simulink model "TestBench"  (Simulink 7.6)
settings: Solver=ode45  StartTime=0.0  StopTime=100  RelTol=1e-3
InitFcn:
  | TestBench_datastruct
  | SCAP
undefined symbols (not defined in the file): determiningBonds, sigbuilder_block
(part 1 of 2)
settings Model: Creator=Zsolt  LastModifiedBy=Zsolt
settings HardwareCC: TargetIntDivRoundTo=Zero  TargetEndianess=LittleEndian  TargetHWDeviceType=MATLAB Host  ProdEqTarget=off
settings RTWCC: SystemTargetFile=rsim.tlc  TemplateMakefile=rsim_default_tmf  Description=Rapid Simulation Target  ProcessScript=rsim_make_rtw_hook
settings RSimTargetCC: TargetFunctionLibrary=ANSI_C  ERTMultiwordTypeDef=System defined  ERTCodeCoverageTool=None  ERTMultiwordLength=256  IsPILTarget=off  EnableShiftOperators=on  PortableWordSizes=off

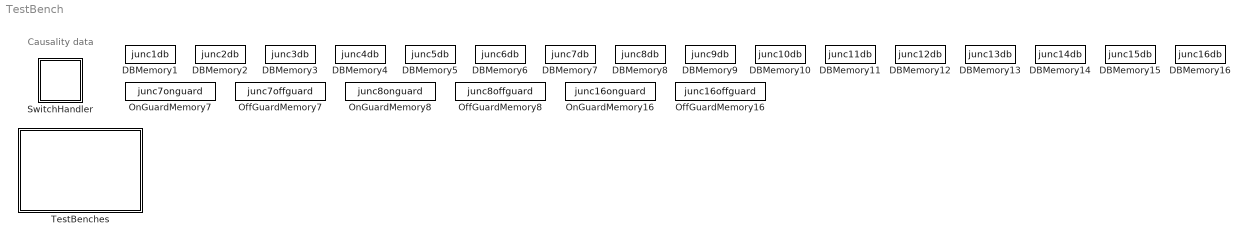
== system TestBench ==
  note: Causality data
  DBMemory1 : DataStoreMemory  DataStoreName=junc1db  InitialValue=determiningBonds(1)
  DBMemory10 : DataStoreMemory  DataStoreName=junc10db  InitialValue=determiningBonds(10)
  DBMemory11 : DataStoreMemory  DataStoreName=junc11db  InitialValue=determiningBonds(11)
  DBMemory12 : DataStoreMemory  DataStoreName=junc12db  InitialValue=determiningBonds(12)
  DBMemory13 : DataStoreMemory  DataStoreName=junc13db  InitialValue=determiningBonds(13)
  DBMemory14 : DataStoreMemory  DataStoreName=junc14db  InitialValue=determiningBonds(14)
  DBMemory15 : DataStoreMemory  DataStoreName=junc15db  InitialValue=determiningBonds(15)
  DBMemory16 : DataStoreMemory  DataStoreName=junc16db  InitialValue=determiningBonds(16)
  DBMemory2 : DataStoreMemory  DataStoreName=junc2db  InitialValue=determiningBonds(2)
  DBMemory3 : DataStoreMemory  DataStoreName=junc3db  InitialValue=determiningBonds(3)
  DBMemory4 : DataStoreMemory  DataStoreName=junc4db  InitialValue=determiningBonds(4)
  DBMemory5 : DataStoreMemory  DataStoreName=junc5db  InitialValue=determiningBonds(5)
  DBMemory6 : DataStoreMemory  DataStoreName=junc6db  InitialValue=determiningBonds(6)
  DBMemory7 : DataStoreMemory  DataStoreName=junc7db  InitialValue=determiningBonds(7)
  DBMemory8 : DataStoreMemory  DataStoreName=junc8db  InitialValue=determiningBonds(8)
  DBMemory9 : DataStoreMemory  DataStoreName=junc9db  InitialValue=determiningBonds(9)
  OffGuardMemory16 : DataStoreMemory  DataStoreName=junc16offguard
  OffGuardMemory7 : DataStoreMemory  DataStoreName=junc7offguard
  OffGuardMemory8 : DataStoreMemory  DataStoreName=junc8offguard
  OnGuardMemory16 : DataStoreMemory  DataStoreName=junc16onguard
  OnGuardMemory7 : DataStoreMemory  DataStoreName=junc7onguard
  OnGuardMemory8 : DataStoreMemory  DataStoreName=junc8onguard
  SwitchHandler : Subsystem
  TestBenches : Subsystem

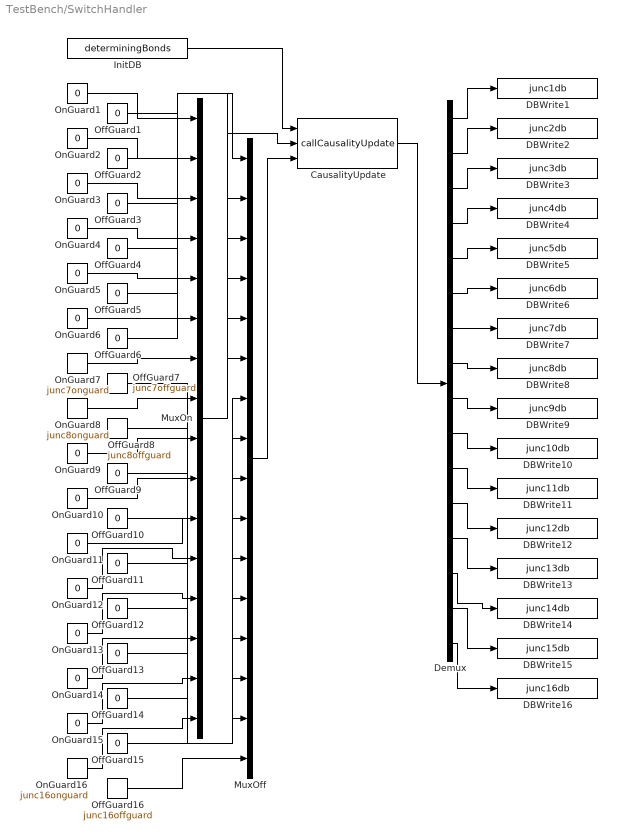
== system TestBench/SwitchHandler ==
  CausalityUpdate : S-Function  FunctionName=callCausalityUpdate  Parameters=16  EnableBusSupport=off
  DBWrite1 : DataStoreWrite  DataStoreName=junc1db
  DBWrite10 : DataStoreWrite  DataStoreName=junc10db
  DBWrite11 : DataStoreWrite  DataStoreName=junc11db
  DBWrite12 : DataStoreWrite  DataStoreName=junc12db
  DBWrite13 : DataStoreWrite  DataStoreName=junc13db
  DBWrite14 : DataStoreWrite  DataStoreName=junc14db
  DBWrite15 : DataStoreWrite  DataStoreName=junc15db
  DBWrite16 : DataStoreWrite  DataStoreName=junc16db
  DBWrite2 : DataStoreWrite  DataStoreName=junc2db
  DBWrite3 : DataStoreWrite  DataStoreName=junc3db
  DBWrite4 : DataStoreWrite  DataStoreName=junc4db
  DBWrite5 : DataStoreWrite  DataStoreName=junc5db
  DBWrite6 : DataStoreWrite  DataStoreName=junc6db
  DBWrite7 : DataStoreWrite  DataStoreName=junc7db
  DBWrite8 : DataStoreWrite  DataStoreName=junc8db
  DBWrite9 : DataStoreWrite  DataStoreName=junc9db
  Demux : Demux  Outputs=16
  InitDB : Constant  Value=determiningBonds
  MuxOff : Mux  Inputs=16
  MuxOn : Mux  Inputs=16
  OffGuard{1..6,9..15} (13 alike) : Constant  Value=0
  OffGuard16 : DataStoreRead  DataStoreName=junc16offguard  SampleTime=0
  OffGuard7 : DataStoreRead  DataStoreName=junc7offguard  SampleTime=0
  OffGuard8 : DataStoreRead  DataStoreName=junc8offguard  SampleTime=0
  OnGuard{1..6,9..15} (13 alike) : Constant  Value=0
  OnGuard16 : DataStoreRead  DataStoreName=junc16onguard  SampleTime=0
  OnGuard7 : DataStoreRead  DataStoreName=junc7onguard  SampleTime=0
  OnGuard8 : DataStoreRead  DataStoreName=junc8onguard  SampleTime=0
  wires:
  OnGuard1/1 -> MuxOn/1
  OffGuard1/1 -> MuxOff/1
  Demux/1 -> DBWrite1/1
  OnGuard2/1 -> MuxOn/2
  OffGuard2/1 -> MuxOff/2
  Demux/2 -> DBWrite2/1
  OnGuard3/1 -> MuxOn/3
  OffGuard3/1 -> MuxOff/3
  Demux/3 -> DBWrite3/1
  OnGuard4/1 -> MuxOn/4
  OffGuard4/1 -> MuxOff/4
  Demux/4 -> DBWrite4/1
  OnGuard5/1 -> MuxOn/5
  OffGuard5/1 -> MuxOff/5
  Demux/5 -> DBWrite5/1
  OnGuard6/1 -> MuxOn/6
  OffGuard6/1 -> MuxOff/6
  Demux/6 -> DBWrite6/1
  OnGuard7/1 -> MuxOn/7
  OffGuard7/1 -> MuxOff/7
  Demux/7 -> DBWrite7/1
  OnGuard8/1 -> MuxOn/8
  OffGuard8/1 -> MuxOff/8
  Demux/8 -> DBWrite8/1
  OnGuard9/1 -> MuxOn/9
  OffGuard9/1 -> MuxOff/9
  Demux/9 -> DBWrite9/1
  OnGuard10/1 -> MuxOn/10
  OffGuard10/1 -> MuxOff/10
  Demux/10 -> DBWrite10/1
  OnGuard11/1 -> MuxOn/11
  OffGuard11/1 -> MuxOff/11
  Demux/11 -> DBWrite11/1
  OnGuard12/1 -> MuxOn/12
  OffGuard12/1 -> MuxOff/12
  Demux/12 -> DBWrite12/1
  OnGuard13/1 -> MuxOn/13
  OffGuard13/1 -> MuxOff/13
  Demux/13 -> DBWrite13/1
  OnGuard14/1 -> MuxOn/14
  OffGuard14/1 -> MuxOff/14
  Demux/14 -> DBWrite14/1
  OnGuard15/1 -> MuxOn/15
  OffGuard15/1 -> MuxOff/15
  Demux/15 -> DBWrite15/1
  OnGuard16/1 -> MuxOn/16
  OffGuard16/1 -> MuxOff/16
  Demux/16 -> DBWrite16/1
  InitDB/1 -> CausalityUpdate/1
  MuxOn/1 -> CausalityUpdate/2
  MuxOff/1 -> CausalityUpdate/3
  CausalityUpdate/1 -> Demux/1

== system TestBench/TestBenches ==
  V_EngISGTest_experiments : Subsystem

== system TestBench/TestBenches/V_EngISGTest_experiments ==
  EngineISG : Subsystem
  RotationalLoad : Subsystem
  ThrottleScenario : Subsystem
  wires:
  EngineISG/1(RotationalPowerPort_1_OUT_5) -> RotationalLoad/1(Rotational Power Port_1_IN_5)
  RotationalLoad/1(Rotational Power Port_1_OUT_5) -> EngineISG/1(RotationalPowerPort_1_IN_5)
  ThrottleScenario/1(Mode) -> EngineISG/5(Mode)
  ThrottleScenario/2(DieselDemand) -> EngineISG/3(Throttle)
  ThrottleScenario/3(ElectDemand) -> EngineISG/4(EP_Demand)

== system TestBench/TestBenches/V_EngISGTest_experiments/EngineISG ==
  RotationalPowerPort_1_IN_5 : Inport
  AddlLoad : Inport  Port=2
  Throttle : Inport  Port=3
  EP_Demand : Inport  Port=4
  Mode : Inport  Port=5
  Battery : Subsystem
  Diesel_Engine : Subsystem
  ISG : Subsystem
  PowerController : Subsystem
  RotationalPowerPort_1_OUT_5 : Outport
  wires:
  Diesel_Engine/1(OutputShaft_1_OUT_2) -> ISG/1(EngSide_1_IN_2)
  ISG/1(EngSide_1_OUT_2) -> Diesel_Engine/1(OutputShaft_1_IN_2)
  Battery/1(Pwr_1_OUT_3) -> PowerController/1(Batt_In_1_IN_3)
  PowerController/1(Batt_In_1_OUT_3) -> Battery/1(Pwr_1_IN_3)
  ISG/2(TransSide_1_OUT_5) -> RotationalPowerPort_1_OUT_5/1
  RotationalPowerPort_1_IN_5/1 -> ISG/2(TransSide_1_IN_5)
  PowerController/2(ISG_Out_1_OUT_7) -> ISG/3(ElectricalPowerPort_1_IN_7)
  ISG/3(ElectricalPowerPort_1_OUT_7) -> PowerController/2(ISG_Out_1_IN_7)
  Throttle/1 -> Diesel_Engine/3(Throttle)
  AddlLoad/1 -> Diesel_Engine/2(Additional_Load)
  Mode/1 -> Battery/2(Mode)
  Battery/2(BatteryVoltage) -> PowerController/4(BattVoltage)
  EP_Demand/1 -> PowerController/5(E_Power_Demand)
  ISG/6(ISG_EngVoltage) -> PowerController/3(ISGVoltage)

== system TestBench/TestBenches/V_EngISGTest_experiments/RotationalLoad ==
  Rotational Power Port_1_IN_5 : Inport
  Load : Constant  Value=3000
  ResistiveLoad : Subsystem
  Targthrottle : Constant
  Rotational Power Port_1_OUT_5 : Outport
  AddLoad : Outport  Port=2
  Throttle : Outport  Port=3
  wires:
  ResistiveLoad/1(MechanicalRPort_1_OUT_5) -> Rotational Power Port_1_OUT_5/1
  Rotational Power Port_1_IN_5/1 -> ResistiveLoad/1(MechanicalRPort_1_IN_5)
  Targthrottle/1 -> Throttle/1
  Load/1 -> AddLoad/1

== system TestBench/TestBenches/V_EngISGTest_experiments/ThrottleScenario ==
  BGDriver : Subsystem
  Mode : Outport
  DieselDemand : Outport  Port=2
  ElectDemand : Outport  Port=3
  wires:
  BGDriver/3(Mode) -> Mode/1
  BGDriver/1(MechPwr) -> DieselDemand/1
  BGDriver/2(ElecPwr) -> ElectDemand/1

== system TestBench/TestBenches/V_EngISGTest_experiments/EngineISG/Battery ==
  Pwr_1_IN_3 : Inport
  Mode : Inport  Port=2
  Battery : Subsystem
  Pwr_1_OUT_3 : Outport
  BatteryVoltage : Outport  Port=2
  wires:
  Battery/1(Pwr_1_OUT_3) -> Pwr_1_OUT_3/1
  Pwr_1_IN_3/1 -> Battery/1(Pwr_1_IN_3)
  Battery/2(Battery_Voltage) -> BatteryVoltage/1
  Mode/1 -> Battery/2(Mode)

== system TestBench/TestBenches/V_EngISGTest_experiments/EngineISG/Diesel_Engine ==
  OutputShaft_1_IN_2 : Inport
  Additional_Load : Inport  Port=2
  Throttle : Inport  Port=3
  Diesel_Engine : Subsystem
  MaxPower : Constant  Value=300000
  MaxTorque : Constant  Value=2000
  OutputShaft_1_OUT_2 : Outport
  Angular_Velocity : Outport  Port=2
  wires:
  Diesel_Engine/1(Out_1_OUT_2) -> OutputShaft_1_OUT_2/1
  OutputShaft_1_IN_2/1 -> Diesel_Engine/1(Out_1_IN_2)
  Diesel_Engine/2(Angular_Velocity) -> Angular_Velocity/1
  Additional_Load/1 -> Diesel_Engine/5(Additional_Load)
  Throttle/1 -> Diesel_Engine/2(Throttle)
  MaxTorque/1 -> Diesel_Engine/3(torqueMax)
  MaxPower/1 -> Diesel_Engine/4(MaxPower)

== system TestBench/TestBenches/V_EngISGTest_experiments/EngineISG/ISG ==
  EngSide_1_IN_2 : Inport
  TransSide_1_IN_5 : Inport  Port=2
  ElectricalPowerPort_1_IN_7 : Inport  Port=3
  ISG_BG : Subsystem
  ISG_Gain : Constant  Value=0.05
  EngSide_1_OUT_2 : Outport
  TransSide_1_OUT_5 : Outport  Port=2
  ElectricalPowerPort_1_OUT_7 : Outport  Port=3
  AngularVelocity : Outport  Port=4
  AddedTorque : Outport  Port=5
  ISG_EngVoltage : Outport  Port=6
  wires:
  ISG_BG/1(EngineSide_1_OUT_2) -> EngSide_1_OUT_2/1
  EngSide_1_IN_2/1 -> ISG_BG/1(EngineSide_1_IN_2)
  ISG_BG/2(TransmissionSide_1_OUT_5) -> TransSide_1_OUT_5/1
  TransSide_1_IN_5/1 -> ISG_BG/2(TransmissionSide_1_IN_5)
  ISG_BG/3(Electrical_1_OUT_7) -> ElectricalPowerPort_1_OUT_7/1
  ElectricalPowerPort_1_IN_7/1 -> ISG_BG/3(Electrical_1_IN_7)
  ISG_BG/4(ISG_AngularVelocity) -> AngularVelocity/1
  ISG_BG/5(ISG_Torque) -> AddedTorque/1
  ISG_BG/6(InV) -> ISG_EngVoltage/1
  ISG_Gain/1 -> ISG_BG/4(ISG_GainInput)

== system TestBench/TestBenches/V_EngISGTest_experiments/EngineISG/PowerController ==
  Batt_In_1_IN_3 : Inport
  ISG_Out_1_IN_7 : Inport  Port=2
  ISGVoltage : Inport  Port=3
  BattVoltage : Inport  Port=4
  E_Power_Demand : Inport  Port=5
  PowerCtrlBG : Subsystem
  Batt_In_1_OUT_3 : Outport
  ISG_Out_1_OUT_7 : Outport  Port=2
  wires:
  PowerCtrlBG/1(Batt_Input_1_OUT_3) -> Batt_In_1_OUT_3/1
  Batt_In_1_IN_3/1 -> PowerCtrlBG/1(Batt_Input_1_IN_3)
  PowerCtrlBG/2(Power_Output_1_OUT_7) -> ISG_Out_1_OUT_7/1
  ISG_Out_1_IN_7/1 -> PowerCtrlBG/2(Power_Output_1_IN_7)
  E_Power_Demand/1 -> PowerCtrlBG/5(Demand)
  BattVoltage/1 -> PowerCtrlBG/4(BattVoltage)
  ISGVoltage/1 -> PowerCtrlBG/3(ISGVoltage)

== system TestBench/TestBenches/V_EngISGTest_experiments/RotationalLoad/ResistiveLoad ==
  MechanicalRPort_1_IN_5 : Inport
  InertialLoad : Subsystem  mask{I=10, IC=0}
      mask prompts: I "Value of I:"; IC "Initial Condition:"
      mask Display: image(imread('I.png','BackgroundColor',[1 1 1]))
  Load_w : Scope
  ResistiveLoad2 : Subsystem  mask{R=1.5}
      mask prompts: R "Value of R:"
      mask Display: image(imread('R.png','BackgroundColor',[1 1 1]))
  Series : Subsystem
      mask Display: image(imread('1.png','BackgroundColor',[1 1 1]))
  zed1 : Subsystem
      mask Display: image(imread('0.png','BackgroundColor',[1 1 1]))
  MechanicalRPort_1_OUT_5 : Outport
  wires:
  zed1/2(y(2)) -> Series/2(u(2))
  Series/2(y(2)) -> zed1/2(u(2))
  Series/1(y(1)) -> ResistiveLoad2/1(In)
  ResistiveLoad2/1(Out) -> Series/1(u(1))
  Series/3(y(3)) -> InertialLoad/1(E)
  InertialLoad/1(F) -> Series/3(u(3))
  zed1/1(y(1)) -> MechanicalRPort_1_OUT_5/1
  MechanicalRPort_1_IN_5/1 -> zed1/1(u(1))
  Series/4(O) -> Load_w/1

== system TestBench/TestBenches/V_EngISGTest_experiments/ThrottleScenario/BGDriver ==
  SimulinkModel : Subsystem
  MechPwr : Outport
  ElecPwr : Outport  Port=2
  Mode : Outport  Port=3
  wires:
  SimulinkModel/1(Mode) -> Mode/1
  SimulinkModel/2(Mech_Pwr) -> MechPwr/1
  SimulinkModel/3(Elect_Pwr) -> ElecPwr/1

== system TestBench/TestBenches/V_EngISGTest_experiments/EngineISG/Battery/Battery ==
  Pwr_1_IN_3 : Inport
  Mode : Inport  Port=2
  C_battery : Subsystem  mask{C=100, IC=24}
      mask prompts: C "Value of C:"; IC "Initial Condition:"
      mask Display: image(imread('C.png','BackgroundColor',[1 1 1]))
  Current_Battery : Scope
  De_batt_voltage : Subsystem  TreatAsAtomicUnit=on
  R_battery : Subsystem  mask{R=0.01}
      mask prompts: R "Value of R:"
      mask Display: image(imread('R.png','BackgroundColor',[1 1 1]))
  Voltage_Battery : Scope
  oj1 : Subsystem
      mask Display: image(imread('1.png','BackgroundColor',[1 1 1]))
  zj2 : Subsystem
      mask Display: image(imread('0.png','BackgroundColor',[1 1 1]))
  Pwr_1_OUT_3 : Outport
  Battery_Voltage : Outport  Port=2
  wires:
  oj1/2(y(2)) -> R_battery/1(In)
  R_battery/1(Out) -> oj1/2(u(2))
  zj2/1(y(1)) -> oj1/3(u(3))
  oj1/3(y(3)) -> zj2/1(u(1))
  zj2/2(y(2)) -> C_battery/1(F)
  C_battery/1(E) -> zj2/2(u(2))
  oj1/1(y(1)) -> Pwr_1_OUT_3/1
  Pwr_1_IN_3/1 -> oj1/1(u(1))
  zj2/3(O) -> Voltage_Battery/1, De_batt_voltage/1(E_In)
  Mode/1 -> oj1/4(u(4))
  De_batt_voltage/1(E_Out) -> Battery_Voltage/1
  oj1/4(O) -> Current_Battery/1

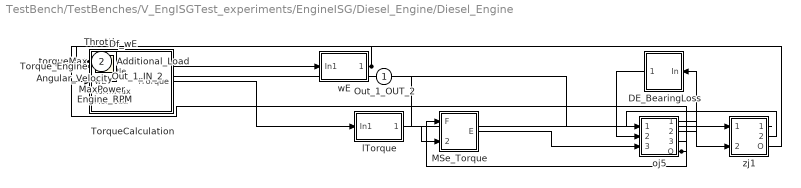
== system TestBench/TestBenches/V_EngISGTest_experiments/EngineISG/Diesel_Engine/Diesel_Engine ==
  Out_1_IN_2 : Inport
  Throttle : Inport  Port=2
  torqueMax : Inport  Port=3
  MaxPower : Inport  Port=4
  Additional_Load : Inport  Port=5
  DE_BearingLoss : Subsystem  mask{R=0.01}
      mask prompts: R "Value of R:"
      mask Display: image(imread('R.png','BackgroundColor',[1 1 1]))
  Df_wE : Subsystem  TreatAsAtomicUnit=on
  Engine_RPM : Scope
  MSe_Torque : Subsystem
      mask Display: image(imread('MSe.png','BackgroundColor',[1 1 1]))
  TorqueCalculation : Stateflow chart  TreatAsAtomicUnit=on
  Torque_Engine : Scope
  lTorque : Subsystem  TreatAsAtomicUnit=on
  oj5 : Subsystem
      mask Display: image(imread('1.png','BackgroundColor',[1 1 1]))
  wE : Subsystem  TreatAsAtomicUnit=on
  zj1 : Subsystem
      mask Display: image(imread('0.png','BackgroundColor',[1 1 1]))
  Out_1_OUT_2 : Outport
  Angular_Velocity : Outport  Port=2
  wires:
  oj5/1(y(1)) -> zj1/2(u(2))
  zj1/2(y(2)) -> oj5/1(u(1))
  oj5/2(y(2)) -> DE_BearingLoss/1(In)
  DE_BearingLoss/1(Out) -> oj5/2(u(2))
  MSe_Torque/1(E) -> oj5/3(u(3))
  oj5/3(y(3)) -> MSe_Torque/1(F)
  zj1/1(y(1)) -> Out_1_OUT_2/1
  Out_1_IN_2/1 -> zj1/1(u(1))
  TorqueCalculation/1(lTorque) -> lTorque/1(In1)
  zj1/3(O) -> Torque_Engine/1
  lTorque/1(Out1) -> MSe_Torque/2(Se Value)
  Throttle/1 -> TorqueCalculation/2(Throttle)
  torqueMax/1 -> TorqueCalculation/4(torqueMax)
  MaxPower/1 -> TorqueCalculation/1(MaxPower)
  Additional_Load/1 -> TorqueCalculation/5(Additional_Load)
  Df_wE/1(F_Out) -> wE/1(In1)
  oj5/4(O) -> Df_wE/1(F_In), Engine_RPM/1
  wE/1(Out1) -> TorqueCalculation/3(wE), Angular_Velocity/1

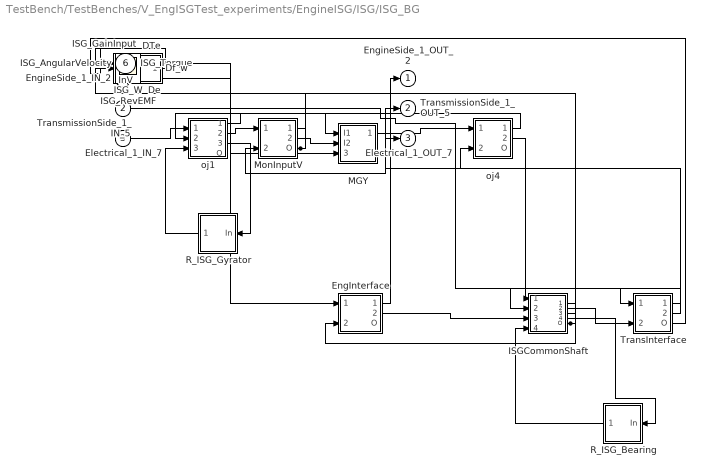
== system TestBench/TestBenches/V_EngISGTest_experiments/EngineISG/ISG/ISG_BG ==
  EngineSide_1_IN_2 : Inport
  TransmissionSide_1_IN_5 : Inport  Port=2
  Electrical_1_IN_7 : Inport  Port=3
  ISG_GainInput : Inport  Port=4
  DTe : Subsystem  TreatAsAtomicUnit=on
  De : Subsystem  TreatAsAtomicUnit=on
  Df_w : Subsystem  TreatAsAtomicUnit=on
  EngInterface : Subsystem
      mask Display: image(imread('0.png','BackgroundColor',[1 1 1]))
  ISGCommonShaft : Subsystem
      mask Display: image(imread('1.png','BackgroundColor',[1 1 1]))
  ISG_RevEMF : Scope
  ISG_W : Scope
  MGY : Subsystem
      mask Display: image(imread('MGY.png','BackgroundColor',[1 1 1]))
  MonInputV : Subsystem
      mask Display: image(imread('0.png','BackgroundColor',[1 1 1]))
  R_ISG_Bearing : Subsystem  mask{R=0.01}
      mask prompts: R "Value of R:"
      mask Display: image(imread('R.png','BackgroundColor',[1 1 1]))
  R_ISG_Gyrator : Subsystem  mask{R=0.01}
      mask prompts: R "Value of R:"
      mask Display: image(imread('R.png','BackgroundColor',[1 1 1]))
  TransInterface : Subsystem
      mask Display: image(imread('0.png','BackgroundColor',[1 1 1]))
  oj1 : Subsystem
      mask Display: image(imread('1.png','BackgroundColor',[1 1 1]))
  oj4 : Subsystem
      mask Display: image(imread('1.png','BackgroundColor',[1 1 1]))
  EngineSide_1_OUT_2 : Outport
  TransmissionSide_1_OUT_5 : Outport  Port=2
  Electrical_1_OUT_7 : Outport  Port=3
  ISG_AngularVelocity : Outport  Port=4
  ISG_Torque : Outport  Port=5
  InV : Outport  Port=6
  wires:
  EngInterface/2(y(2)) -> ISGCommonShaft/3(u(3))
  ISGCommonShaft/3(y(3)) -> EngInterface/2(u(2))
  oj1/2(y(2)) -> MonInputV/1(u(1))
  MonInputV/1(y(1)) -> oj1/2(u(2))
  oj1/3(y(3)) -> R_ISG_Gyrator/1(In)
  R_ISG_Gyrator/1(Out) -> oj1/3(u(3))
  MGY/1(O1) -> oj4/1(u(1))
  oj4/1(y(1)) -> MGY/1(I1)
  oj4/2(y(2)) -> ISGCommonShaft/1(u(1))
  ISGCommonShaft/1(y(1)) -> oj4/2(u(2))
  ISGCommonShaft/2(y(2)) -> TransInterface/2(u(2))
  TransInterface/2(y(2)) -> ISGCommonShaft/2(u(2))
  ISGCommonShaft/4(y(4)) -> R_ISG_Bearing/1(In)
  R_ISG_Bearing/1(Out) -> ISGCommonShaft/4(u(4))
  MonInputV/2(y(2)) -> MGY/2(I2)
  MGY/2(O2) -> MonInputV/2(u(2))
  EngInterface/1(y(1)) -> EngineSide_1_OUT_2/1
  EngineSide_1_IN_2/1 -> EngInterface/1(u(1))
  TransInterface/1(y(1)) -> TransmissionSide_1_OUT_5/1
  TransmissionSide_1_IN_5/1 -> TransInterface/1(u(1))
  oj1/1(y(1)) -> Electrical_1_OUT_7/1
  Electrical_1_IN_7/1 -> oj1/1(u(1))
  Df_w/1(F_Out) -> ISG_AngularVelocity/1
  TransInterface/3(O) -> De/1(E_In)
  ISGCommonShaft/5(O) -> Df_w/1(F_In), ISG_W/1
  De/1(E_Out) -> ISG_Torque/1
  DTe/1(E_Out) -> InV/1
  MonInputV/3(O) -> DTe/1(E_In), ISG_RevEMF/1
  ISG_GainInput/1 -> MGY/3(GY Value)

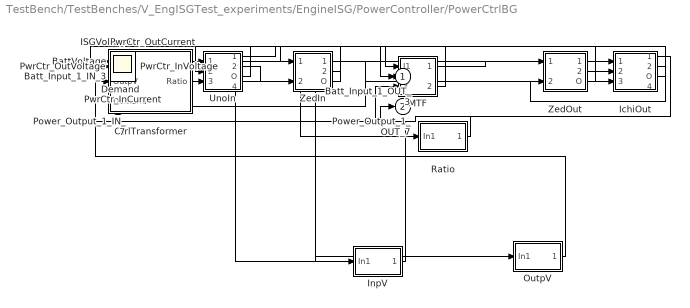
== system TestBench/TestBenches/V_EngISGTest_experiments/EngineISG/PowerController/PowerCtrlBG ==
  Batt_Input_1_IN_3 : Inport
  Power_Output_1_IN_7 : Inport  Port=2
  ISGVoltage : Inport  Port=3
  BattVoltage : Inport  Port=4
  Demand : Inport  Port=5
  CtrlTransformer : Stateflow chart  TreatAsAtomicUnit=on
  IchiOut : Subsystem
      mask Display: image(imread('1.png','BackgroundColor',[1 1 1]))
  InpV : Subsystem  TreatAsAtomicUnit=on
  MTF : Subsystem
      mask Display: image(imread('MTF.png','BackgroundColor',[1 1 1]))
  OutpV : Subsystem  TreatAsAtomicUnit=on
  PwrCtr_InCurrent : Scope
  PwrCtr_InVoltage : Scope
  PwrCtr_OutCurrent : Scope
  PwrCtr_OutVoltage : Scope
  Ratio : Subsystem  TreatAsAtomicUnit=on
  UnoIn : Subsystem
      mask Display: image(imread('1.png','BackgroundColor',[1 1 1]))
  ZedIn : Subsystem
      mask Display: image(imread('0.png','BackgroundColor',[1 1 1]))
  ZedOut : Subsystem
      mask Display: image(imread('0.png','BackgroundColor',[1 1 1]))
  Batt_Input_1_OUT_3 : Outport
  Power_Output_1_OUT_7 : Outport  Port=2
  wires:
  UnoIn/2(y(2)) -> ZedIn/2(u(2))
  ZedIn/2(y(2)) -> UnoIn/2(u(2))
  MTF/1(O1) -> ZedOut/1(u(1))
  ZedOut/1(y(1)) -> MTF/1(I1)
  ZedOut/2(y(2)) -> IchiOut/2(u(2))
  IchiOut/2(y(2)) -> ZedOut/2(u(2))
  ZedIn/1(y(1)) -> MTF/2(I2)
  MTF/2(O2) -> ZedIn/1(u(1))
  UnoIn/1(y(1)) -> Batt_Input_1_OUT_3/1
  Batt_Input_1_IN_3/1 -> UnoIn/1(u(1))
  IchiOut/1(y(1)) -> Power_Output_1_OUT_7/1
  Power_Output_1_IN_7/1 -> IchiOut/1(u(1))
  ISGVoltage/1 -> OutpV/1(In1)
  BattVoltage/1 -> InpV/1(In1)
  InpV/1(Out1) -> CtrlTransformer/1(InpV)
  UnoIn/3(O) -> PwrCtr_InCurrent/1
  Demand/1 -> UnoIn/3(u(3)), IchiOut/3(u(3)), CtrlTransformer/3(Demand)
  ZedIn/3(O) -> PwrCtr_InVoltage/1
  OutpV/1(Out1) -> CtrlTransformer/2(OutpV)
  IchiOut/3(O) -> PwrCtr_OutCurrent/1
  ZedOut/3(O) -> PwrCtr_OutVoltage/1
  Ratio/1(Out1) -> MTF/3(TF Value)
  CtrlTransformer/1(Ratio) -> Ratio/1(In1)

== system TestBench/TestBenches/V_EngISGTest_experiments/RotationalLoad/ResistiveLoad/InertialLoad ==
  E : Inport
  Inductance : Constant  Value=I
  InitialCondition : Constant  Value=IC
  Initialization : InitialCondition  Value=IC
  Integrator : Integrator  InitialConditionSource=external
  Product1 : Product  SaturateOnIntegerOverflow=on  RndMeth=Zero  InputSameDT=on  OutDataTypeStr=Inherit: Same as first input
  Product2 : Product  SaturateOnIntegerOverflow=on  RndMeth=Zero  InputSameDT=on  OutDataTypeStr=Inherit: Same as first input
  Reciprocal : Math  Operator=reciprocal  SaturateOnIntegerOverflow=on
  F : Outport
  p : Outport  Port=2
  wires:
  E/1 -> Integrator/1
  InitialCondition/1 -> Initialization/1
  Initialization/1 -> Product1/1
  Inductance/1 -> Reciprocal/1, Product1/2
  Product1/1 -> Integrator/2
  Integrator/1 -> Product2/1, p/1
  Reciprocal/1 -> Product2/2
  Product2/1 -> F/1

== system TestBench/TestBenches/V_EngISGTest_experiments/RotationalLoad/ResistiveLoad/ResistiveLoad2 ==
  In : Inport
  Bond : Constant
  Computing R : Subsystem
  JuncDB : Constant  Value=3
  Junction Type : Constant
  Resistor Value : Constant  Value=R
  Out : Outport
  wires:
  In/1 -> Computing R/1(In1)
  Resistor Value/1 -> Computing R/2(R)
  JuncDB/1 -> Computing R/3(JuncDB)
  Bond/1 -> Computing R/4(Bond)
  Junction Type/1 -> Computing R/5(Junction Type)
  Computing R/1(Out1) -> Out/1

== system TestBench/TestBenches/V_EngISGTest_experiments/RotationalLoad/ResistiveLoad/Series ==
  u(1) : Inport
  u(2) : Inport  Port=2
  u(3) : Inport  Port=3
  Adder : Sum  Inputs=+-  SaturateOnIntegerOverflow=on  InputSameDT=on  OutDataTypeStr=Inherit: Same as first input
  Gain : Gain  Gain=-1  SaturateOnIntegerOverflow=on  OutDataTypeStr=Inherit: Same as input  ParamDataTypeStr=Inherit: Same as input
  y(1) : Outport
  y(2) : Outport  Port=2
  y(3) : Outport  Port=3
  O : Outport  Port=4
  wires:
  Adder/1 -> Gain/1
  u(3)/1 -> y(1)/1, y(2)/1, O/1
  u(1)/1 -> Adder/1
  u(2)/1 -> Adder/2
  Gain/1 -> y(3)/1

== system TestBench/TestBenches/V_EngISGTest_experiments/RotationalLoad/ResistiveLoad/zed1 ==
  u(1) : Inport
  u(2) : Inport  Port=2
  Adder : Sum  Inputs=+  SaturateOnIntegerOverflow=on  InputSameDT=on  OutDataTypeStr=Inherit: Same as first input
  Gain : Gain  SaturateOnIntegerOverflow=on  OutDataTypeStr=Inherit: Same as input  ParamDataTypeStr=Inherit: Same as input
  y(1) : Outport
  y(2) : Outport  Port=2
  O : Outport  Port=3
  wires:
  Adder/1 -> Gain/1
  Gain/1 -> y(1)/1
  u(1)/1 -> y(2)/1, O/1
  u(2)/1 -> Adder/1

== system TestBench/TestBenches/V_EngISGTest_experiments/ThrottleScenario/BGDriver/SimulinkModel ==
  Mode Signal Builder : Subsystem  Tag=STV Subsys  LoadFcn=sigbuilder_block('load');  StartFcn=sigbuilder_block('start');  StopFcn=sigbuilder_block('stop');  ClipboardFcn=sigbuilder_block('clipboard');  mask(Sigbuilder block){}
      mask help: Create and generate interchangeable groups of signals whose waveforms are piecewise linear.
      mask init:
      | if ~strcmp(get_param(bdroot(gcbh),'SimulationStatus'),'stopped') tuvar = sigbuilder_block('maskInit'); end
      settings: CopyFcn=sigbuilder_block('copy');  DeleteFcn=sigbuilder_block('delete');  ModelCloseFcn=sigbuilder_block('modelClose');  PreSaveFcn=sigbuilder_block('preSave');  NameChangeFcn=sigbuilder_block('namechange');  OpenFcn=sigbuilder_block('open',[215.25 65.25 852.75 489.75 ]);  CloseFcn=sigbuilder_block('close');
      mask Display: plot(0,0,100,100,[10,10,40,40,10],[80,20,20,80,80],[40,10],[50,50], [40,27,10],[65,72,56],[40,25,25,10],[28,28,43,43]);
  Zsolt version : Subsystem  Tag=STV Subsys  LoadFcn=sigbuilder_block('load');  StartFcn=sigbuilder_block('start');  StopFcn=sigbuilder_block('stop');  ClipboardFcn=sigbuilder_block('clipboard');  mask(Sigbuilder block){}
      mask help: Create and generate interchangeable groups of signals whose waveforms are piecewise linear.
      mask init:
      | if ~strcmp(get_param(bdroot(gcbh),'SimulationStatus'),'stopped') tuvar = sigbuilder_block('maskInit'); end
      settings: CopyFcn=sigbuilder_block('copy');  DeleteFcn=sigbuilder_block('delete');  ModelCloseFcn=sigbuilder_block('modelClose');  PreSaveFcn=sigbuilder_block('preSave');  NameChangeFcn=sigbuilder_block('namechange');  OpenFcn=sigbuilder_block('open',[9 35.25 852.75 281.25 ]);  CloseFcn=sigbuilder_block('close');
      mask Display: plot(0,0,100,100,[10,10,40,40,10],[80,20,20,80,80],[40,10],[50,50], [40,27,10],[65,72,56],[40,25,25,10],[28,28,43,43]);
  Mode : Outport
  Mech_Pwr : Outport  Port=2
  Elect_Pwr : Outport  Port=3
  wires:
  Zsolt version/1(Mode) -> Mode/1
  Zsolt version/2(Mech_Pwr) -> Mech_Pwr/1
  Zsolt version/3(Elect_Pwr) -> Elect_Pwr/1

== system TestBench/TestBenches/V_EngISGTest_experiments/EngineISG/Battery/Battery/C_battery ==
  F : Inport
  Capacitance : Constant  Value=C
  InitialCondition : Constant  Value=IC
  Initialization : InitialCondition  Value=IC
  Integrator : Integrator  InitialConditionSource=external
  Product1 : Product  SaturateOnIntegerOverflow=on  RndMeth=Zero  InputSameDT=on  OutDataTypeStr=Inherit: Same as first input
  Product2 : Product  SaturateOnIntegerOverflow=on  RndMeth=Zero  InputSameDT=on  OutDataTypeStr=Inherit: Same as first input
  Reciprocal : Math  Operator=reciprocal  SaturateOnIntegerOverflow=on
  E : Outport
  q : Outport  Port=2
  wires:
  F/1 -> Integrator/1
  InitialCondition/1 -> Initialization/1
  Initialization/1 -> Product1/1
  Capacitance/1 -> Reciprocal/1, Product1/2
  Product1/1 -> Integrator/2
  Integrator/1 -> Product2/1, q/1
  Reciprocal/1 -> Product2/2
  Product2/1 -> E/1

== system TestBench/TestBenches/V_EngISGTest_experiments/EngineISG/Battery/Battery/De_batt_voltage ==
  E_In : Inport
  E_Out : Outport
  wires:
  E_In/1 -> E_Out/1

== system TestBench/TestBenches/V_EngISGTest_experiments/EngineISG/Battery/Battery/R_battery ==
  In : Inport
  Bond : Constant  Value=2
  Computing R : Subsystem
  JuncDB : DataStoreRead  DataStoreName=junc7db  SampleTime=0
  Junction Type : Constant
  Resistor Value : Constant  Value=R
  Out : Outport
  wires:
  In/1 -> Computing R/1(In1)
  Resistor Value/1 -> Computing R/2(R)
  JuncDB/1 -> Computing R/3(JuncDB)
  Bond/1 -> Computing R/4(Bond)
  Junction Type/1 -> Computing R/5(Junction Type)
  Computing R/1(Out1) -> Out/1

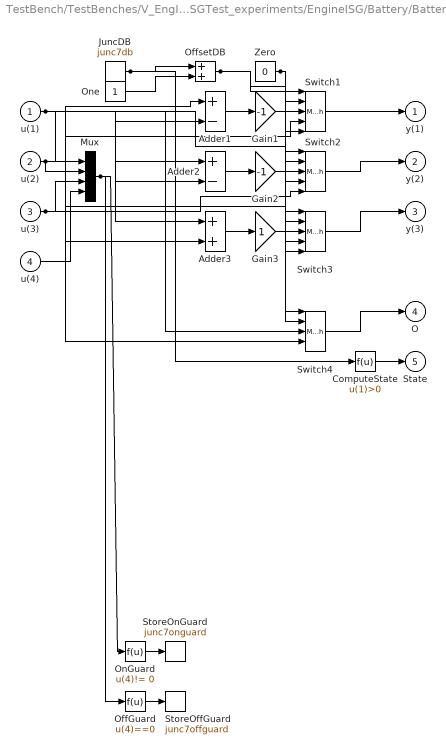
== system TestBench/TestBenches/V_EngISGTest_experiments/EngineISG/Battery/Battery/oj1 ==
  u(1) : Inport
  u(2) : Inport  Port=2
  u(3) : Inport  Port=3
  u(4) : Inport  Port=4
  Adder1 : Sum  Inputs=+-  SaturateOnIntegerOverflow=on  InputSameDT=on  OutDataTypeStr=Inherit: Same as first input
  Adder2 : Sum  Inputs=+-  SaturateOnIntegerOverflow=on  InputSameDT=on  OutDataTypeStr=Inherit: Same as first input
  Adder3 : Sum  SaturateOnIntegerOverflow=on  InputSameDT=on  OutDataTypeStr=Inherit: Same as first input
  ComputeState : Fcn  Expr=u(1)>0
  Gain1 : Gain  Gain=-1  SaturateOnIntegerOverflow=on  OutDataTypeStr=Inherit: Same as input  ParamDataTypeStr=Inherit: Same as input
  Gain2 : Gain  Gain=-1  SaturateOnIntegerOverflow=on  OutDataTypeStr=Inherit: Same as input  ParamDataTypeStr=Inherit: Same as input
  Gain3 : Gain  SaturateOnIntegerOverflow=on  OutDataTypeStr=Inherit: Same as input  ParamDataTypeStr=Inherit: Same as input
  JuncDB : DataStoreRead  DataStoreName=junc7db  SampleTime=0
  Mux : Mux
  OffGuard : Fcn  Expr=u(4)==0
  OffsetDB : Sum  SaturateOnIntegerOverflow=on  InputSameDT=on  OutDataTypeStr=Inherit: Same as first input
  OnGuard : Fcn  Expr=u(4)!= 0
  One : Constant
  StoreOffGuard : DataStoreWrite  DataStoreName=junc7offguard
  StoreOnGuard : DataStoreWrite  DataStoreName=junc7onguard
  Switch{1..4} (4 alike) : MultiPortSwitch  Inputs=4  zeroidx=off  SaturateOnIntegerOverflow=on  InputSameDT=on
  Zero : Constant  Value=0
  y(1) : Outport
  y(2) : Outport  Port=2
  y(3) : Outport  Port=3
  O : Outport  Port=4
  State : Outport  Port=5
  wires:
  JuncDB/1 -> OffsetDB/1, ComputeState/1
  One/1 -> OffsetDB/2
  Switch1/1 -> y(1)/1
  OffsetDB/1 -> Switch1/1, Switch2/1, Switch3/1, Switch4/1
  Zero/1 -> Switch1/2, Switch2/2, Switch3/2, Switch4/2
  Adder1/1 -> Gain1/1
  u(1)/1 -> Mux/1, Switch2/3, Adder2/1, Switch3/3, Adder3/1, Switch4/3
  Switch2/1 -> y(2)/1
  Adder2/1 -> Gain2/1
  u(2)/1 -> Mux/2, Switch1/4, Adder1/1, Switch3/4, Adder3/2, Switch4/4
  Switch3/1 -> y(3)/1
  Adder3/1 -> Gain3/1
  u(3)/1 -> Mux/3, Switch1/5, Adder1/2, Switch2/5, Adder2/2
  Switch4/1 -> O/1
  ComputeState/1 -> State/1
  Gain1/1 -> Switch1/3
  Gain2/1 -> Switch2/4
  Gain3/1 -> Switch3/5
  u(4)/1 -> Mux/4
  Mux/1 -> OnGuard/1, OffGuard/1
  OnGuard/1 -> StoreOnGuard/1
  OffGuard/1 -> StoreOffGuard/1

== system TestBench/TestBenches/V_EngISGTest_experiments/EngineISG/Battery/Battery/zj2 ==
  u(1) : Inport
  u(2) : Inport  Port=2
  Adder : Sum  Inputs=+  SaturateOnIntegerOverflow=on  InputSameDT=on  OutDataTypeStr=Inherit: Same as first input
  Gain : Gain  Gain=-1  SaturateOnIntegerOverflow=on  OutDataTypeStr=Inherit: Same as input  ParamDataTypeStr=Inherit: Same as input
  y(1) : Outport
  y(2) : Outport  Port=2
  O : Outport  Port=3
  wires:
  Adder/1 -> Gain/1
  u(2)/1 -> y(1)/1, O/1
  u(1)/1 -> Adder/1
  Gain/1 -> y(2)/1

== system TestBench/TestBenches/V_EngISGTest_experiments/EngineISG/Diesel_Engine/Diesel_Engine/DE_BearingLoss ==
  In : Inport
  Bond : Constant  Value=2
  Computing R : Subsystem
  JuncDB : Constant
  Junction Type : Constant
  Resistor Value : Constant  Value=R
  Out : Outport
  wires:
  In/1 -> Computing R/1(In1)
  Resistor Value/1 -> Computing R/2(R)
  JuncDB/1 -> Computing R/3(JuncDB)
  Bond/1 -> Computing R/4(Bond)
  Junction Type/1 -> Computing R/5(Junction Type)
  Computing R/1(Out1) -> Out/1

== system TestBench/TestBenches/V_EngISGTest_experiments/EngineISG/Diesel_Engine/Diesel_Engine/Df_wE ==
  F_In : Inport
  F_Out : Outport
  wires:
  F_In/1 -> F_Out/1

== system TestBench/TestBenches/V_EngISGTest_experiments/EngineISG/Diesel_Engine/Diesel_Engine/MSe_Torque ==
  F : Inport
  Se Value : Inport  Port=2
  E : Outport
  wires:
  Se Value/1 -> E/1

== system TestBench/TestBenches/V_EngISGTest_experiments/EngineISG/Diesel_Engine/Diesel_Engine/lTorque ==
  In1 : Inport
  Out1 : Outport
  wires:
  In1/1 -> Out1/1

== system TestBench/TestBenches/V_EngISGTest_experiments/EngineISG/Diesel_Engine/Diesel_Engine/oj5 ==
  u(1) : Inport
  u(2) : Inport  Port=2
  u(3) : Inport  Port=3
  Adder : Sum  Inputs=+-  SaturateOnIntegerOverflow=on  InputSameDT=on  OutDataTypeStr=Inherit: Same as first input
  Gain : Gain  Gain=-1  SaturateOnIntegerOverflow=on  OutDataTypeStr=Inherit: Same as input  ParamDataTypeStr=Inherit: Same as input
  y(1) : Outport
  y(2) : Outport  Port=2
  y(3) : Outport  Port=3
  O : Outport  Port=4
  wires:
  Adder/1 -> Gain/1
  Gain/1 -> y(1)/1
  u(1)/1 -> y(2)/1, y(3)/1, O/1
  u(2)/1 -> Adder/1
  u(3)/1 -> Adder/2

== system TestBench/TestBenches/V_EngISGTest_experiments/EngineISG/Diesel_Engine/Diesel_Engine/wE ==
  In1 : Inport
  Out1 : Outport
  wires:
  In1/1 -> Out1/1

== system TestBench/TestBenches/V_EngISGTest_experiments/EngineISG/Diesel_Engine/Diesel_Engine/zj1 ==
  u(1) : Inport
  u(2) : Inport  Port=2
  Adder : Sum  Inputs=+  SaturateOnIntegerOverflow=on  InputSameDT=on  OutDataTypeStr=Inherit: Same as first input
  Gain : Gain  SaturateOnIntegerOverflow=on  OutDataTypeStr=Inherit: Same as input  ParamDataTypeStr=Inherit: Same as input
  y(1) : Outport
  y(2) : Outport  Port=2
  O : Outport  Port=3
  wires:
  Adder/1 -> Gain/1
  u(2)/1 -> y(1)/1, O/1
  u(1)/1 -> Adder/1
  Gain/1 -> y(2)/1

== system TestBench/TestBenches/V_EngISGTest_experiments/EngineISG/ISG/ISG_BG/DTe ==
  E_In : Inport
  E_Out : Outport
  wires:
  E_In/1 -> E_Out/1

== system TestBench/TestBenches/V_EngISGTest_experiments/EngineISG/ISG/ISG_BG/De ==
  E_In : Inport
  E_Out : Outport
  wires:
  E_In/1 -> E_Out/1

== system TestBench/TestBenches/V_EngISGTest_experiments/EngineISG/ISG/ISG_BG/Df_w ==
  F_In : Inport
  F_Out : Outport
  wires:
  F_In/1 -> F_Out/1

== system TestBench/TestBenches/V_EngISGTest_experiments/EngineISG/ISG/ISG_BG/EngInterface ==
  u(1) : Inport
  u(2) : Inport  Port=2
  Adder : Sum  Inputs=+  SaturateOnIntegerOverflow=on  InputSameDT=on  OutDataTypeStr=Inherit: Same as first input
  Gain : Gain  SaturateOnIntegerOverflow=on  OutDataTypeStr=Inherit: Same as input  ParamDataTypeStr=Inherit: Same as input
  y(1) : Outport
  y(2) : Outport  Port=2
  O : Outport  Port=3
  wires:
  Adder/1 -> Gain/1
  Gain/1 -> y(1)/1
  u(1)/1 -> y(2)/1, O/1
  u(2)/1 -> Adder/1

== system TestBench/TestBenches/V_EngISGTest_experiments/EngineISG/ISG/ISG_BG/ISGCommonShaft ==
  u(1) : Inport
  u(2) : Inport  Port=2
  u(3) : Inport  Port=3
  u(4) : Inport  Port=4
  Adder : Sum  Inputs=--+  SaturateOnIntegerOverflow=on  InputSameDT=on  OutDataTypeStr=Inherit: Same as first input
  Gain : Gain  Gain=-1  SaturateOnIntegerOverflow=on  OutDataTypeStr=Inherit: Same as input  ParamDataTypeStr=Inherit: Same as input
  y(1) : Outport
  y(2) : Outport  Port=2
  y(3) : Outport  Port=3
  y(4) : Outport  Port=4
  O : Outport  Port=5
  wires:
  Adder/1 -> Gain/1
  u(2)/1 -> y(1)/1, y(3)/1, y(4)/1, O/1
  u(1)/1 -> Adder/1
  Gain/1 -> y(2)/1
  u(3)/1 -> Adder/2
  u(4)/1 -> Adder/3

== system TestBench/TestBenches/V_EngISGTest_experiments/EngineISG/ISG/ISG_BG/MGY ==
  I1 : Inport
  I2 : Inport  Port=2
  GY Value : Inport  Port=3
  Gain1 : Product  SaturateOnIntegerOverflow=on  RndMeth=Zero  InputSameDT=on  OutDataTypeStr=Inherit: Same as first input
  Gain2 : Product  SaturateOnIntegerOverflow=on  RndMeth=Zero  InputSameDT=on  OutDataTypeStr=Inherit: Same as first input
  O1 : Outport
  O2 : Outport  Port=2
  wires:
  I1/1 -> Gain1/1
  I2/1 -> Gain2/1
  GY Value/1 -> Gain1/2, Gain2/2
  Gain1/1 -> O2/1
  Gain2/1 -> O1/1

== system TestBench/TestBenches/V_EngISGTest_experiments/EngineISG/ISG/ISG_BG/MonInputV ==
  u(1) : Inport
  u(2) : Inport  Port=2
  Adder : Sum  Inputs=-  SaturateOnIntegerOverflow=on  InputSameDT=on  OutDataTypeStr=Inherit: Same as first input
  Gain : Gain  Gain=-1  SaturateOnIntegerOverflow=on  OutDataTypeStr=Inherit: Same as input  ParamDataTypeStr=Inherit: Same as input
  y(1) : Outport
  y(2) : Outport  Port=2
  O : Outport  Port=3
  wires:
  Adder/1 -> Gain/1
  u(2)/1 -> y(1)/1, O/1
  u(1)/1 -> Adder/1
  Gain/1 -> y(2)/1

== system TestBench/TestBenches/V_EngISGTest_experiments/EngineISG/ISG/ISG_BG/R_ISG_Bearing ==
  In : Inport
  Bond : Constant  Value=4
  Computing R : Subsystem
  JuncDB : Constant  Value=2
  Junction Type : Constant
  Resistor Value : Constant  Value=R
  Out : Outport
  wires:
  In/1 -> Computing R/1(In1)
  Resistor Value/1 -> Computing R/2(R)
  JuncDB/1 -> Computing R/3(JuncDB)
  Bond/1 -> Computing R/4(Bond)
  Junction Type/1 -> Computing R/5(Junction Type)
  Computing R/1(Out1) -> Out/1

== system TestBench/TestBenches/V_EngISGTest_experiments/EngineISG/ISG/ISG_BG/R_ISG_Gyrator ==
  In : Inport
  Bond : Constant  Value=3
  Computing R : Subsystem
  JuncDB : DataStoreRead  DataStoreName=junc9db  SampleTime=0
  Junction Type : Constant
  Resistor Value : Constant  Value=R
  Out : Outport
  wires:
  In/1 -> Computing R/1(In1)
  Resistor Value/1 -> Computing R/2(R)
  JuncDB/1 -> Computing R/3(JuncDB)
  Bond/1 -> Computing R/4(Bond)
  Junction Type/1 -> Computing R/5(Junction Type)
  Computing R/1(Out1) -> Out/1

== system TestBench/TestBenches/V_EngISGTest_experiments/EngineISG/ISG/ISG_BG/TransInterface ==
  u(1) : Inport
  u(2) : Inport  Port=2
  Adder : Sum  Inputs=+  SaturateOnIntegerOverflow=on  InputSameDT=on  OutDataTypeStr=Inherit: Same as first input
  Gain : Gain  SaturateOnIntegerOverflow=on  OutDataTypeStr=Inherit: Same as input  ParamDataTypeStr=Inherit: Same as input
  y(1) : Outport
  y(2) : Outport  Port=2
  O : Outport  Port=3
  wires:
  Adder/1 -> Gain/1
  u(2)/1 -> y(1)/1, O/1
  u(1)/1 -> Adder/1
  Gain/1 -> y(2)/1

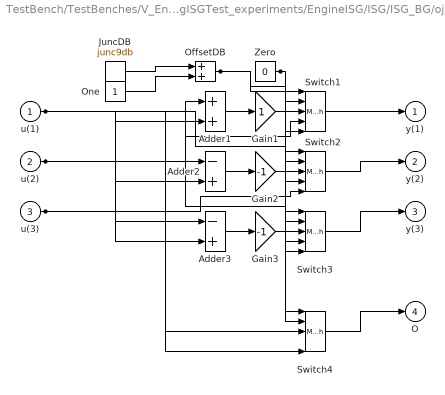
== system TestBench/TestBenches/V_EngISGTest_experiments/EngineISG/ISG/ISG_BG/oj1 ==
  u(1) : Inport
  u(2) : Inport  Port=2
  u(3) : Inport  Port=3
  Adder1 : Sum  SaturateOnIntegerOverflow=on  InputSameDT=on  OutDataTypeStr=Inherit: Same as first input
  Adder2 : Sum  Inputs=-+  SaturateOnIntegerOverflow=on  InputSameDT=on  OutDataTypeStr=Inherit: Same as first input
  Adder3 : Sum  Inputs=-+  SaturateOnIntegerOverflow=on  InputSameDT=on  OutDataTypeStr=Inherit: Same as first input
  Gain1 : Gain  SaturateOnIntegerOverflow=on  OutDataTypeStr=Inherit: Same as input  ParamDataTypeStr=Inherit: Same as input
  Gain2 : Gain  Gain=-1  SaturateOnIntegerOverflow=on  OutDataTypeStr=Inherit: Same as input  ParamDataTypeStr=Inherit: Same as input
  Gain3 : Gain  Gain=-1  SaturateOnIntegerOverflow=on  OutDataTypeStr=Inherit: Same as input  ParamDataTypeStr=Inherit: Same as input
  JuncDB : DataStoreRead  DataStoreName=junc9db  SampleTime=0
  OffsetDB : Sum  SaturateOnIntegerOverflow=on  InputSameDT=on  OutDataTypeStr=Inherit: Same as first input
  One : Constant
  Switch{1..4} (4 alike) : MultiPortSwitch  Inputs=4  zeroidx=off  SaturateOnIntegerOverflow=on  InputSameDT=on
  Zero : Constant  Value=0
  y(1) : Outport
  y(2) : Outport  Port=2
  y(3) : Outport  Port=3
  O : Outport  Port=4
  wires:
  JuncDB/1 -> OffsetDB/1
  One/1 -> OffsetDB/2
  Switch1/1 -> y(1)/1
  OffsetDB/1 -> Switch1/1, Switch2/1, Switch3/1, Switch4/1
  Zero/1 -> Switch1/2, Switch2/2, Switch3/2, Switch4/2
  Adder1/1 -> Gain1/1
  Switch2/1 -> y(2)/1
  Adder2/1 -> Gain2/1
  Switch3/1 -> y(3)/1
  Adder3/1 -> Gain3/1
  Switch4/1 -> O/1
  Gain1/1 -> Switch1/3
  u(1)/1 -> Switch2/3, Adder2/1, Switch3/3, Adder3/1, Switch4/3
  u(2)/1 -> Switch1/4, Adder1/1, Switch3/4, Adder3/2
  Gain2/1 -> Switch2/4
  u(3)/1 -> Switch1/5, Adder1/2, Switch2/5, Adder2/2, Switch4/5
  Gain3/1 -> Switch3/5

== system TestBench/TestBenches/V_EngISGTest_experiments/EngineISG/ISG/ISG_BG/oj4 ==
  u(1) : Inport
  u(2) : Inport  Port=2
  Adder : Sum  Inputs=-  SaturateOnIntegerOverflow=on  InputSameDT=on  OutDataTypeStr=Inherit: Same as first input
  Gain : Gain  Gain=-1  SaturateOnIntegerOverflow=on  OutDataTypeStr=Inherit: Same as input  ParamDataTypeStr=Inherit: Same as input
  y(1) : Outport
  y(2) : Outport  Port=2
  O : Outport  Port=3
  wires:
  Adder/1 -> Gain/1
  u(2)/1 -> y(1)/1, O/1
  u(1)/1 -> Adder/1
  Gain/1 -> y(2)/1

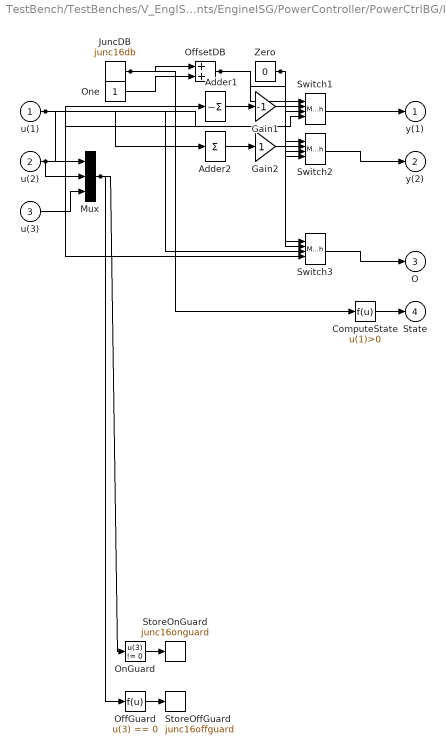
== system TestBench/TestBenches/V_EngISGTest_experiments/EngineISG/PowerController/PowerCtrlBG/IchiOut ==
  u(1) : Inport
  u(2) : Inport  Port=2
  u(3) : Inport  Port=3
  Adder1 : Sum  Inputs=-  SaturateOnIntegerOverflow=on  InputSameDT=on  OutDataTypeStr=Inherit: Same as first input
  Adder2 : Sum  Inputs=+  SaturateOnIntegerOverflow=on  InputSameDT=on  OutDataTypeStr=Inherit: Same as first input
  ComputeState : Fcn  Expr=u(1)>0
  Gain1 : Gain  Gain=-1  SaturateOnIntegerOverflow=on  OutDataTypeStr=Inherit: Same as input  ParamDataTypeStr=Inherit: Same as input
  Gain2 : Gain  SaturateOnIntegerOverflow=on  OutDataTypeStr=Inherit: Same as input  ParamDataTypeStr=Inherit: Same as input
  JuncDB : DataStoreRead  DataStoreName=junc16db  SampleTime=0
  Mux : Mux  Inputs=3
  OffGuard : Fcn  Expr=u(3) == 0
  OffsetDB : Sum  SaturateOnIntegerOverflow=on  InputSameDT=on  OutDataTypeStr=Inherit: Same as first input
  OnGuard : Fcn  Expr=u(3) != 0
  One : Constant
  StoreOffGuard : DataStoreWrite  DataStoreName=junc16offguard
  StoreOnGuard : DataStoreWrite  DataStoreName=junc16onguard
  Switch1 : MultiPortSwitch  zeroidx=off  SaturateOnIntegerOverflow=on  InputSameDT=on
  Switch2 : MultiPortSwitch  zeroidx=off  SaturateOnIntegerOverflow=on  InputSameDT=on
  Switch3 : MultiPortSwitch  zeroidx=off  SaturateOnIntegerOverflow=on  InputSameDT=on
  Zero : Constant  Value=0
  y(1) : Outport
  y(2) : Outport  Port=2
  O : Outport  Port=3
  State : Outport  Port=4
  wires:
  JuncDB/1 -> OffsetDB/1, ComputeState/1
  One/1 -> OffsetDB/2
  Switch1/1 -> y(1)/1
  OffsetDB/1 -> Switch1/1, Switch2/1, Switch3/1
  Zero/1 -> Switch1/2, Switch2/2, Switch3/2
  Adder1/1 -> Gain1/1
  u(1)/1 -> Mux/1, Switch2/3, Adder2/1, Switch3/3
  Switch2/1 -> y(2)/1
  Adder2/1 -> Gain2/1
  u(2)/1 -> Mux/2, Switch1/4, Adder1/1, Switch3/4
  Switch3/1 -> O/1
  ComputeState/1 -> State/1
  Gain1/1 -> Switch1/3
  Gain2/1 -> Switch2/4
  u(3)/1 -> Mux/3
  Mux/1 -> OnGuard/1, OffGuard/1
  OnGuard/1 -> StoreOnGuard/1
  OffGuard/1 -> StoreOffGuard/1

== system TestBench/TestBenches/V_EngISGTest_experiments/EngineISG/PowerController/PowerCtrlBG/InpV ==
  In1 : Inport
  Out1 : Outport
  wires:
  In1/1 -> Out1/1

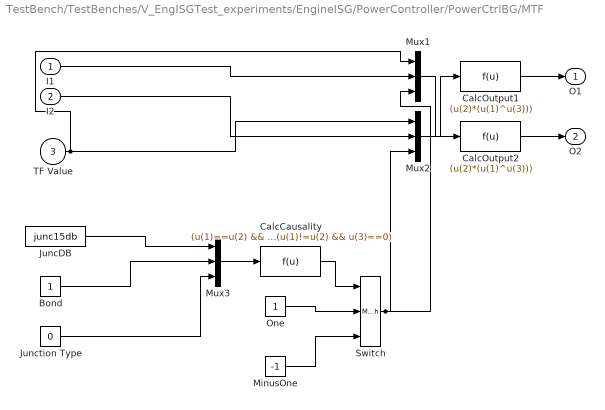
== system TestBench/TestBenches/V_EngISGTest_experiments/EngineISG/PowerController/PowerCtrlBG/MTF ==
  I1 : Inport
  I2 : Inport  Port=2
  TF Value : Inport  Port=3
  Bond : Constant
  CalcCausality : Fcn  Expr=(u(1)==u(2) && u(3)==1) || (u(1)!=u(2) && u(3)==0)
  CalcOutput1 : Fcn  Expr=(u(2)*(u(1)^u(3)))
  CalcOutput2 : Fcn  Expr=(u(2)*(u(1)^u(3)))
  JuncDB : DataStoreRead  DataStoreName=junc15db
  Junction Type : Constant  Value=0
  MinusOne : Constant  Value=-1
  Mux1 : Mux  Inputs=3
  Mux2 : Mux  Inputs=3
  Mux3 : Mux  Inputs=3
  One : Constant
  Switch : MultiPortSwitch  DataPortOrder=Zero-based contiguous  Inputs=2  zeroidx=on  SaturateOnIntegerOverflow=on  InputSameDT=on
  O1 : Outport
  O2 : Outport  Port=2
  wires:
  I1/1 -> Mux1/2
  I2/1 -> Mux2/2
  TF Value/1 -> Mux1/1, Mux2/1
  Switch/1 -> Mux1/3, Mux2/3
  JuncDB/1 -> Mux3/1
  Bond/1 -> Mux3/2
  Junction Type/1 -> Mux3/3
  Mux1/1 -> CalcOutput2/1
  Mux2/1 -> CalcOutput1/1
  Mux3/1 -> CalcCausality/1
  CalcCausality/1 -> Switch/1
  One/1 -> Switch/2
  MinusOne/1 -> Switch/3
  CalcOutput1/1 -> O1/1
  CalcOutput2/1 -> O2/1

== system TestBench/TestBenches/V_EngISGTest_experiments/EngineISG/PowerController/PowerCtrlBG/OutpV ==
  In1 : Inport
  Out1 : Outport
  wires:
  In1/1 -> Out1/1

== system TestBench/TestBenches/V_EngISGTest_experiments/EngineISG/PowerController/PowerCtrlBG/Ratio ==
  In1 : Inport
  Out1 : Outport
  wires:
  In1/1 -> Out1/1

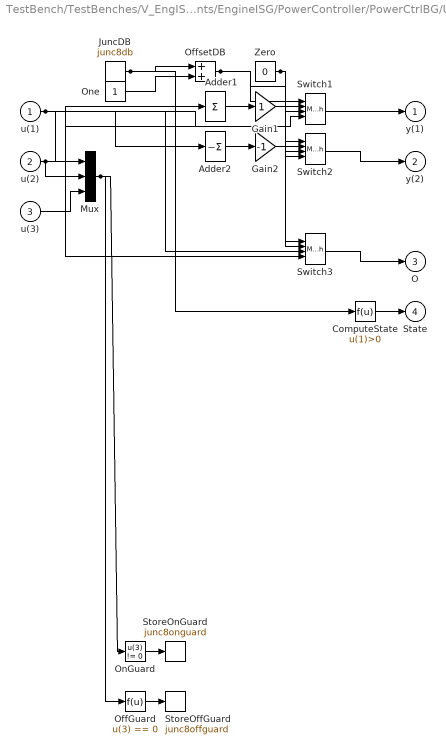
== system TestBench/TestBenches/V_EngISGTest_experiments/EngineISG/PowerController/PowerCtrlBG/UnoIn ==
  u(1) : Inport
  u(2) : Inport  Port=2
  u(3) : Inport  Port=3
  Adder1 : Sum  Inputs=+  SaturateOnIntegerOverflow=on  InputSameDT=on  OutDataTypeStr=Inherit: Same as first input
  Adder2 : Sum  Inputs=-  SaturateOnIntegerOverflow=on  InputSameDT=on  OutDataTypeStr=Inherit: Same as first input
  ComputeState : Fcn  Expr=u(1)>0
  Gain1 : Gain  SaturateOnIntegerOverflow=on  OutDataTypeStr=Inherit: Same as input  ParamDataTypeStr=Inherit: Same as input
  Gain2 : Gain  Gain=-1  SaturateOnIntegerOverflow=on  OutDataTypeStr=Inherit: Same as input  ParamDataTypeStr=Inherit: Same as input
  JuncDB : DataStoreRead  DataStoreName=junc8db  SampleTime=0
  Mux : Mux  Inputs=3
  OffGuard : Fcn  Expr=u(3) == 0
  OffsetDB : Sum  SaturateOnIntegerOverflow=on  InputSameDT=on  OutDataTypeStr=Inherit: Same as first input
  OnGuard : Fcn  Expr=u(3) != 0
  One : Constant
  StoreOffGuard : DataStoreWrite  DataStoreName=junc8offguard
  StoreOnGuard : DataStoreWrite  DataStoreName=junc8onguard
  Switch1 : MultiPortSwitch  zeroidx=off  SaturateOnIntegerOverflow=on  InputSameDT=on
  Switch2 : MultiPortSwitch  zeroidx=off  SaturateOnIntegerOverflow=on  InputSameDT=on
  Switch3 : MultiPortSwitch  zeroidx=off  SaturateOnIntegerOverflow=on  InputSameDT=on
  Zero : Constant  Value=0
  y(1) : Outport
  y(2) : Outport  Port=2
  O : Outport  Port=3
  State : Outport  Port=4
  wires:
  JuncDB/1 -> OffsetDB/1, ComputeState/1
  One/1 -> OffsetDB/2
  Switch1/1 -> y(1)/1
  OffsetDB/1 -> Switch1/1, Switch2/1, Switch3/1
  Zero/1 -> Switch1/2, Switch2/2, Switch3/2
  Adder1/1 -> Gain1/1
  u(1)/1 -> Mux/1, Switch2/3, Adder2/1, Switch3/3
  Switch2/1 -> y(2)/1
  Adder2/1 -> Gain2/1
  u(2)/1 -> Mux/2, Switch1/4, Adder1/1, Switch3/4
  Switch3/1 -> O/1
  ComputeState/1 -> State/1
  Gain1/1 -> Switch1/3
  Gain2/1 -> Switch2/4
  u(3)/1 -> Mux/3
  Mux/1 -> OnGuard/1, OffGuard/1
  OnGuard/1 -> StoreOnGuard/1
  OffGuard/1 -> StoreOffGuard/1

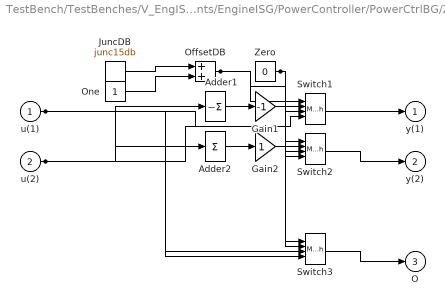
== system TestBench/TestBenches/V_EngISGTest_experiments/EngineISG/PowerController/PowerCtrlBG/ZedIn ==
  u(1) : Inport
  u(2) : Inport  Port=2
  Adder1 : Sum  Inputs=-  SaturateOnIntegerOverflow=on  InputSameDT=on  OutDataTypeStr=Inherit: Same as first input
  Adder2 : Sum  Inputs=+  SaturateOnIntegerOverflow=on  InputSameDT=on  OutDataTypeStr=Inherit: Same as first input
  Gain1 : Gain  Gain=-1  SaturateOnIntegerOverflow=on  OutDataTypeStr=Inherit: Same as input  ParamDataTypeStr=Inherit: Same as input
  Gain2 : Gain  SaturateOnIntegerOverflow=on  OutDataTypeStr=Inherit: Same as input  ParamDataTypeStr=Inherit: Same as input
  JuncDB : DataStoreRead  DataStoreName=junc15db  SampleTime=0
  OffsetDB : Sum  SaturateOnIntegerOverflow=on  InputSameDT=on  OutDataTypeStr=Inherit: Same as first input
  One : Constant
  Switch1 : MultiPortSwitch  zeroidx=off  SaturateOnIntegerOverflow=on  InputSameDT=on
  Switch2 : MultiPortSwitch  zeroidx=off  SaturateOnIntegerOverflow=on  InputSameDT=on
  Switch3 : MultiPortSwitch  zeroidx=off  SaturateOnIntegerOverflow=on  InputSameDT=on
  Zero : Constant  Value=0
  y(1) : Outport
  y(2) : Outport  Port=2
  O : Outport  Port=3
  wires:
  JuncDB/1 -> OffsetDB/1
  One/1 -> OffsetDB/2
  Switch1/1 -> y(1)/1
  OffsetDB/1 -> Switch1/1, Switch2/1, Switch3/1
  Zero/1 -> Switch1/2, Switch2/2, Switch3/2
  Adder1/1 -> Gain1/1
  Switch2/1 -> y(2)/1
  Adder2/1 -> Gain2/1
  Switch3/1 -> O/1
  Gain1/1 -> Switch1/3
  u(1)/1 -> Switch2/3, Adder2/1, Switch3/3
  u(2)/1 -> Switch1/4, Adder1/1, Switch3/4
  Gain2/1 -> Switch2/4

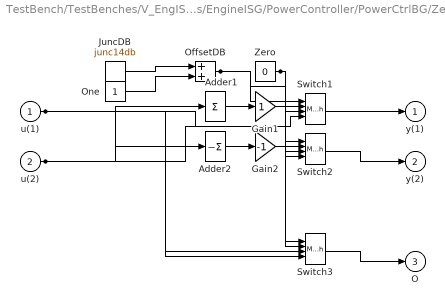
== system TestBench/TestBenches/V_EngISGTest_experiments/EngineISG/PowerController/PowerCtrlBG/ZedOut ==
  u(1) : Inport
  u(2) : Inport  Port=2
  Adder1 : Sum  Inputs=+  SaturateOnIntegerOverflow=on  InputSameDT=on  OutDataTypeStr=Inherit: Same as first input
  Adder2 : Sum  Inputs=-  SaturateOnIntegerOverflow=on  InputSameDT=on  OutDataTypeStr=Inherit: Same as first input
  Gain1 : Gain  SaturateOnIntegerOverflow=on  OutDataTypeStr=Inherit: Same as input  ParamDataTypeStr=Inherit: Same as input
  Gain2 : Gain  Gain=-1  SaturateOnIntegerOverflow=on  OutDataTypeStr=Inherit: Same as input  ParamDataTypeStr=Inherit: Same as input
  JuncDB : DataStoreRead  DataStoreName=junc14db  SampleTime=0
  OffsetDB : Sum  SaturateOnIntegerOverflow=on  InputSameDT=on  OutDataTypeStr=Inherit: Same as first input
  One : Constant
  Switch1 : MultiPortSwitch  zeroidx=off  SaturateOnIntegerOverflow=on  InputSameDT=on
  Switch2 : MultiPortSwitch  zeroidx=off  SaturateOnIntegerOverflow=on  InputSameDT=on
  Switch3 : MultiPortSwitch  zeroidx=off  SaturateOnIntegerOverflow=on  InputSameDT=on
  Zero : Constant  Value=0
  y(1) : Outport
  y(2) : Outport  Port=2
  O : Outport  Port=3
  wires:
  JuncDB/1 -> OffsetDB/1
  One/1 -> OffsetDB/2
  Switch1/1 -> y(1)/1
  OffsetDB/1 -> Switch1/1, Switch2/1, Switch3/1
  Zero/1 -> Switch1/2, Switch2/2, Switch3/2
  Adder1/1 -> Gain1/1
  Switch2/1 -> y(2)/1
  Adder2/1 -> Gain2/1
  Switch3/1 -> O/1
  Gain1/1 -> Switch1/3
  u(1)/1 -> Switch2/3, Adder2/1, Switch3/3
  u(2)/1 -> Switch1/4, Adder1/1, Switch3/4
  Gain2/1 -> Switch2/4

== system TestBench/TestBenches/V_EngISGTest_experiments/RotationalLoad/ResistiveLoad/ResistiveLoad2/Computing R ==
  In1 : Inport
  R : Inport  Port=2
  JuncDB : Inport  Port=3
  Bond : Inport  Port=4
  Junction Type : Inport  Port=5
  CalcCausality : Fcn  Expr=(u(1) == u(2) && u(3) ==1) || (u(1) !=u(2) && u(3) == 0)
  CalcOutput : Fcn  Expr=(u(1)*u(2)^u(3))
  MinusOne : Constant  Value=-1
  Mux1 : Mux  Inputs=3
  Mux2 : Mux  Inputs=3
  One : Constant
  Switch1 : MultiPortSwitch  DataPortOrder=Zero-based contiguous  Inputs=2  zeroidx=on  SaturateOnIntegerOverflow=on  InputSameDT=on
  Out1 : Outport
  wires:
  In1/1 -> Mux2/1
  R/1 -> Mux2/2
  JuncDB/1 -> Mux1/1
  Bond/1 -> Mux1/2
  Junction Type/1 -> Mux1/3
  Mux1/1 -> CalcCausality/1
  CalcCausality/1 -> Switch1/1
  One/1 -> Switch1/2
  MinusOne/1 -> Switch1/3
  Switch1/1 -> Mux2/3
  Mux2/1 -> CalcOutput/1
  CalcOutput/1 -> Out1/1

== system TestBench/TestBenches/V_EngISGTest_experiments/ThrottleScenario/BGDriver/SimulinkModel/Mode Signal Builder ==
  Demux : Demux  Tag=STV Demux  Outputs=3
  FromWs : FromWorkspace  Tag=STV FromWs  VariableName=tuvar  SampleTime=0  SigBuilderData=DataTag0  VnvData=DataTag1
      SigBuilderData=|
      | common.afterFinalStr = 'Extrapolate'
      | common.sampleTime = 0
      | dataSet.timeRange = [0 1000]
      | dataSet.name = 'Group 1'
      | sbobj.Groups.Name = 'Group 1'
      | sbobj.Groups.Signals(1).Name = 'Mode'
      | sbobj.Groups.Signals(1).XData = [0 62 62 398 1000]
      | sbobj.Groups.Signals(1).YData = [1 1 0 0 0]
      | sbobj.Groups.Signals(2).Name = 'Mech_Pwr'
      | sbobj.Groups.Signals(2).XData = [0 16 16 239 239 1000]
      | sbobj.Groups.Signals(2).YData = [0.58 0.58 0.24 0.24 0.44 0.44]
      | sbobj.Groups.Signals(3).Name = 'Elect_Pwr'
      | sbobj.Groups.Signals(3).XData = [0 16 16 44 44 60 60 81 81 1000]
      | sbobj.Groups.Signals(3).YData = [37 37 -32.5 -32.5 -0.5 -0.5 -1 -1 -1 -1]
      | sbobj.Groups.TimeRange = [0 1000]
  Mode : Outport  Tag=STV Outport
  Mech_Pwr : Outport  Tag=STV Outport  Port=2
  Elect_Pwr : Outport  Tag=STV Outport  Port=3
  wires:
  Demux/1 -> Mode/1
  FromWs/1 -> Demux/1
  Demux/2 -> Mech_Pwr/1
  Demux/3 -> Elect_Pwr/1

== system TestBench/TestBenches/V_EngISGTest_experiments/ThrottleScenario/BGDriver/SimulinkModel/Zsolt version ==
  Demux : Demux  Tag=STV Demux  Outputs=3
  FromWs : FromWorkspace  Tag=STV FromWs  VariableName=tuvar  SampleTime=0  SigBuilderData=DataTag2  VnvData=DataTag3
      SigBuilderData=|
      | common.afterFinalStr = 'Extrapolate'
      | common.sampleTime = 0
      | dataSet.timeRange = [0 100]
      | dataSet.name = 'Group 1'
      | sbobj.Groups.Name = 'Group 1'
      | sbobj.Groups.Signals(1).Name = 'Mode'
      | sbobj.Groups.Signals(1).XData = [0 43.3 43.3 62 62 100]
      | sbobj.Groups.Signals(1).YData = [1 1 0 0 1 1]
      | sbobj.Groups.Signals(2).Name = 'Mech_Pwr'
      | sbobj.Groups.Signals(2).XData = [0 15.1 15.1 100]
      | sbobj.Groups.Signals(2).YData = [0.68 0.68 0.24 0.24]
      | sbobj.Groups.Signals(3).Name = 'Elect_Pwr'
      | sbobj.Groups.Signals(3).XData = [0 2 2 60 60 77.2 77.2 78.8 78.8 100]
      | sbobj.Groups.Signals(3).YData = [40 40 5 5 -80 -80 30 30 -15 -15]
      | sbobj.Groups.TimeRange = [0 100]
  Mode : Outport  Tag=STV Outport
  Mech_Pwr : Outport  Tag=STV Outport  Port=2
  Elect_Pwr : Outport  Tag=STV Outport  Port=3
  wires:
  Demux/3 -> Elect_Pwr/1
  Demux/2 -> Mech_Pwr/1
  FromWs/1 -> Demux/1
  Demux/1 -> Mode/1

== system TestBench/TestBenches/V_EngISGTest_experiments/EngineISG/Battery/Battery/R_battery/Computing R ==
  In1 : Inport
  R : Inport  Port=2
  JuncDB : Inport  Port=3
  Bond : Inport  Port=4
  Junction Type : Inport  Port=5
  CalcCausality : Fcn  Expr=(u(1) == u(2) && u(3) ==1) || (u(1) !=u(2) && u(3) == 0)
  CalcOutput : Fcn  Expr=(u(1)*u(2)^u(3))
  MinusOne : Constant  Value=-1
  Mux1 : Mux  Inputs=3
  Mux2 : Mux  Inputs=3
  One : Constant
  Switch1 : MultiPortSwitch  DataPortOrder=Zero-based contiguous  Inputs=2  zeroidx=on  SaturateOnIntegerOverflow=on  InputSameDT=on
  Out1 : Outport
  wires:
  In1/1 -> Mux2/1
  R/1 -> Mux2/2
  JuncDB/1 -> Mux1/1
  Bond/1 -> Mux1/2
  Junction Type/1 -> Mux1/3
  Mux1/1 -> CalcCausality/1
  CalcCausality/1 -> Switch1/1
  One/1 -> Switch1/2
  MinusOne/1 -> Switch1/3
  Switch1/1 -> Mux2/3
  Mux2/1 -> CalcOutput/1
  CalcOutput/1 -> Out1/1
